simulink model "EDGE_DETECTOR"  (R2016b)
settings: Solver=VariableStepAuto  StartTime=0.0  StopTime=0.05  RelTol=1e-3
settings Model: Creator=AKSHAY JP PAWAR  LastModifiedBy=AKSHAY JP PAWAR
settings DataIOCC: ReturnWorkspaceOutputs=on
settings SFSimCC: SimUseLocalCustomCode=on
settings RTWCC: RTWUseLocalCustomCode=on

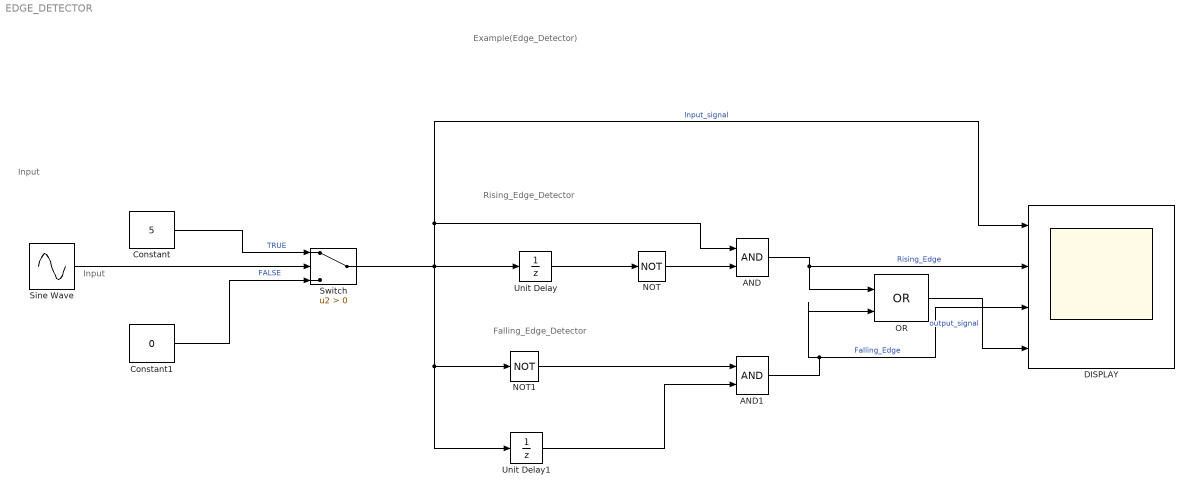
== system EDGE_DETECTOR ==
  note: Input
  note: Example(Edge_Detector)
  note: Falling_Edge_Detector
  note: Rising_Edge_Detector
  note: Input
  AND : Logic  IconShape=distinctive  AllPortsSameDT=off  OutDataTypeStr=boolean
  AND1 : Logic  IconShape=distinctive  AllPortsSameDT=off  OutDataTypeStr=boolean
  Constant : Constant  Value=5
  Constant1 : Constant  Value=0
  DISPLAY : Scope  NumInputPorts=4
  NOT : Logic  Operator=NOT  IconShape=distinctive  AllPortsSameDT=off  OutDataTypeStr=boolean
  NOT1 : Logic  Operator=NOT  IconShape=distinctive  AllPortsSameDT=off  OutDataTypeStr=boolean
  OR : Logic  Operator=OR  IconShape=distinctive  AllPortsSameDT=off  OutDataTypeStr=boolean
  Sine Wave : Sin  Amplitude=5  Frequency=314  SampleTime=0
  Switch : Switch  Criteria=u2 > Threshold
  Unit Delay : UnitDelay  SampleTime=-1  HasFrameUpgradeWarning=on
  Unit Delay1 : UnitDelay  SampleTime=-1  HasFrameUpgradeWarning=on
  wires:
  Unit Delay/1 -> NOT/1
  NOT1/1 -> AND1/1
  Unit Delay1/1 -> AND1/2
  Constant/1 -> Switch/1  "TRUE"
  Constant1/1 -> Switch/3  "FALSE"
  Sine Wave/1 -> Switch/2
  NOT/1 -> AND/2
  Switch/1 -> DISPLAY/1, AND/1, Unit Delay1/1, NOT1/1, Unit Delay/1  "Input_signal"
  AND/1 -> OR/1, DISPLAY/2  "Rising_Edge"
  AND1/1 -> DISPLAY/3, OR/2  "Falling_Edge"
  OR/1 -> DISPLAY/4  "output_signal"
